simulink model "anotherTestModel"  (R2019b)
settings: Solver=FixedStepAuto  StartTime=0.0  StopTime=10.0  FixedStep=.1  RelTol=1e-3
libraries: FaultDetector x2, simulink x1
settings Model: Creator=Nick  LastModifiedBy=Nick

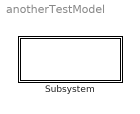
== system anotherTestModel ==
  Subsystem : Subsystem

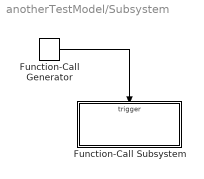
== system anotherTestModel/Subsystem ==
  Function-Call Generator : simulink/Ports & Subsystems/Function-Call Generator  sample_time=.1  numberOfIterations=1
  Function-Call Subsystem : Subsystem  TreatAsAtomicUnit=on
  wires:
  Function-Call Generator/1 -> Function-Call Subsystem/Trigger

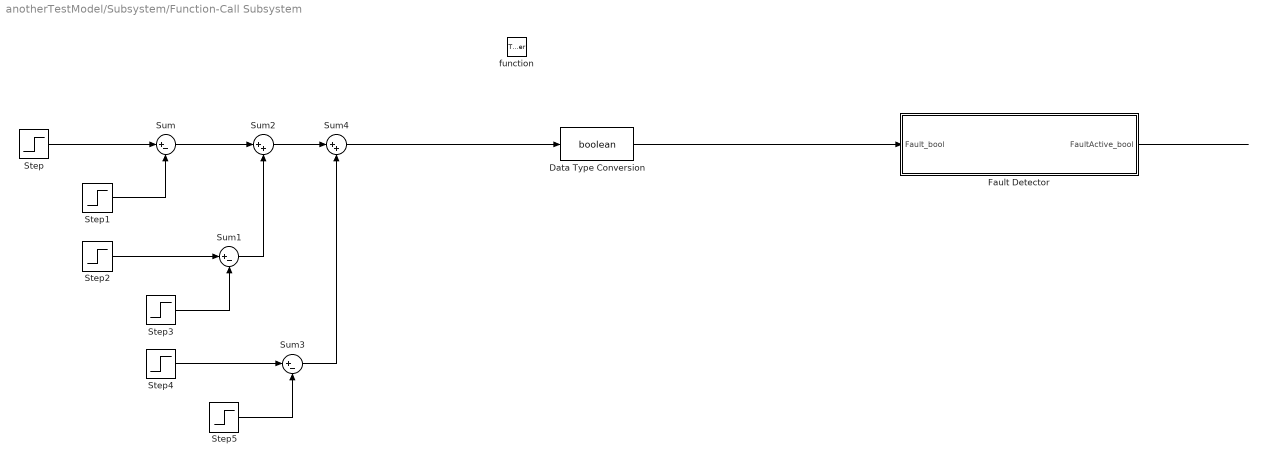
== system anotherTestModel/Subsystem/Function-Call Subsystem ==
  function : TriggerPort  TriggerType=function-call  VariantControl=Variant
  Data Type Conversion : DataTypeConversion  OutDataTypeStr=boolean
  Fault Detector : Subsystem  mask{timeTrip=0, timeReset=0, isSticky=off}
      mask prompts: timeTrip "Time to Trip (s):"; timeReset "Time to Reset (s):"; isSticky "Sticky Fault"
      mask Display:
      | color('blue');
      | 
      | prompt = 'Fault Detector';
      | 
      | if (isSticky)
      |     prompt = [prompt, '\n(Sticky)'];
      |     prompt = [prompt, '\nTrip Time: ', num2str(timeTrip), 's'];
      | else
      |     prompt = [prompt, '\n(Resettable)'];
      |     prompt = [prompt, '\nTrip Time: ', num2str(timeTrip), 's'];
      |     prompt = [prompt, '\nReset Time: ', num2str(timeReset), 's'];
      | end
      | 
      | 
      | 
      | disp(sprintf(prompt));
  Step : Step  Time=5
  Step1 : Step  Time=5.5
  Step2 : Step  Time=6
  Step3 : Step  Time=6.5
  Step4 : Step  Time=7
  Step5 : Step  Time=7.5
  Sum : Sum  Inputs=|+-
  Sum1 : Sum  Inputs=|+-
  Sum2 : Sum  Inputs=|++
  Sum3 : Sum  Inputs=|+-
  Sum4 : Sum  Inputs=|++
  wires:
  Step/1 -> Sum/1
  Data Type Conversion/1 -> Fault Detector/1(Fault_bool)
  Sum/1 -> Sum2/1
  Step1/1 -> Sum/2
  Step2/1 -> Sum1/1
  Step3/1 -> Sum1/2
  Sum2/1 -> Sum4/1
  Sum1/1 -> Sum2/2
  Step5/1 -> Sum3/2
  Step4/1 -> Sum3/1
  Sum4/1 -> Data Type Conversion/1
  Sum3/1 -> Sum4/2
  Fault Detector/1(FaultActive_bool) -> ?

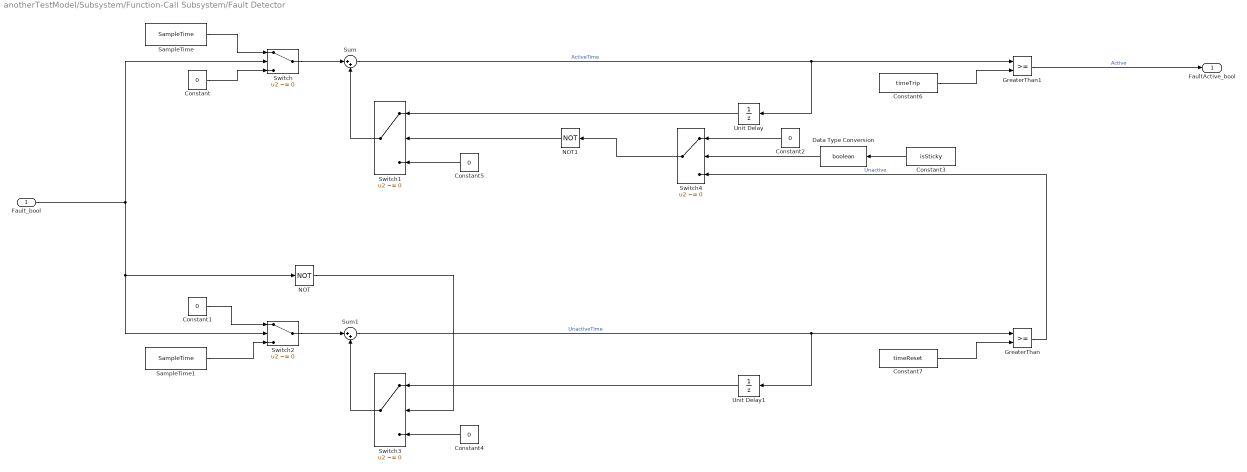
== system anotherTestModel/Subsystem/Function-Call Subsystem/Fault Detector ==
  Fault_bool : Inport  OutDataTypeStr=boolean
  Constant{,1..2,4..5} (5 alike) : Constant  Value=0
  Constant3 : Constant  Value=isSticky
  Constant6 : Constant  Value=timeTrip
  Constant7 : Constant  Value=timeReset
  Data Type Conversion : DataTypeConversion  OutDataTypeStr=boolean
  GreaterThan : RelationalOperator  OutDataTypeStr=boolean  RndMeth=Simplest
  GreaterThan1 : RelationalOperator  OutDataTypeStr=boolean  RndMeth=Simplest
  NOT : Logic  Operator=NOT  IconShape=distinctive  AllPortsSameDT=off  OutDataTypeStr=boolean
  NOT1 : Logic  Operator=NOT  IconShape=distinctive  AllPortsSameDT=off  OutDataTypeStr=boolean
  SampleTime : FaultDetector/Algroithms/SampleTime  SystemSampleTime=-1  SSRTWFcnClass=[]  Latency=0  AutoFrameSizeCalculation=off
  SampleTime1 : FaultDetector/Algroithms/SampleTime  SystemSampleTime=-1  SSRTWFcnClass=[]  Latency=0  AutoFrameSizeCalculation=off
  Sum : Sum  Inputs=|++
  Sum1 : Sum  Inputs=|++
  Switch{,1..4} (5 alike) : Switch  Criteria=u2 ~= 0
  Unit Delay : UnitDelay  SampleTime=-1  HasFrameUpgradeWarning=on
  Unit Delay1 : UnitDelay  SampleTime=-1  HasFrameUpgradeWarning=on
  FaultActive_bool : Outport  OutDataTypeStr=boolean
  wires:
  Switch/1 -> Sum/1
  SampleTime/1 -> Switch/1
  Constant/1 -> Switch/3
  Switch1/1 -> Sum/2
  Sum/1 -> GreaterThan1/1, Unit Delay/1  "ActiveTime"
  Unit Delay/1 -> Switch1/1
  Sum1/1 -> GreaterThan/1, Unit Delay1/1  "UnactiveTime"
  Unit Delay1/1 -> Switch3/1
  Constant1/1 -> Switch2/1
  Switch2/1 -> Sum1/1
  Switch3/1 -> Sum1/2
  SampleTime1/1 -> Switch2/3
  NOT/1 -> Switch3/2
  Constant7/1 -> GreaterThan/2
  Constant6/1 -> GreaterThan1/2
  GreaterThan1/1 -> FaultActive_bool/1  "Active"
  GreaterThan/1 -> Switch4/3  "Unactive"
  Constant4/1 -> Switch3/3
  Constant5/1 -> Switch1/3
  NOT1/1 -> Switch1/2
  Fault_bool/1 -> NOT/1, Switch2/2, Switch/2
  Switch4/1 -> NOT1/1
  Constant2/1 -> Switch4/1
  Constant3/1 -> Data Type Conversion/1
  Data Type Conversion/1 -> Switch4/2
